simulink model "Cart_Pendulum_n9558292"  (R2018a)
settings: Solver=VariableStepAuto  StartTime=0.0  StopTime=10.0  RelTol=1e-3
model workspace (MAT data in the model file):
  F = 5
values from neighbouring files (symbols this model uses):
  g = 9.81    [MainFile_Linearised_a_n9558292.m]    (also in MainFile_Linearised_b_n9558292.m; MainFile_n9558292.m)
  l = 0.2    [MainFile_Linearised_a_n9558292.m]    (also in MainFile_Linearised_b_n9558292.m; MainFile_n9558292.m)
  m = 0.15    [MainFile_Linearised_a_n9558292.m]    (also in MainFile_Linearised_b_n9558292.m; MainFile_n9558292.m)
  Mc = 0.4    [MainFile_Linearised_a_n9558292.m]    (also in MainFile_Linearised_b_n9558292.m; MainFile_n9558292.m)
  stepf = 0.1    [MainFile_n9558292.m]
  stepi = 0    [MainFile_n9558292.m]
  stept = 1    [MainFile_n9558292.m]
  x10 = 0    [MainFile_n9558292.m]
  x20 = pi    (= 3.14159265359)    [MainFile_n9558292.m]
  x30 = 0    [MainFile_n9558292.m]
  x40 = 0    [MainFile_n9558292.m]
settings Model: Creator=haidarobeid  LastModifiedBy=haidarobeid

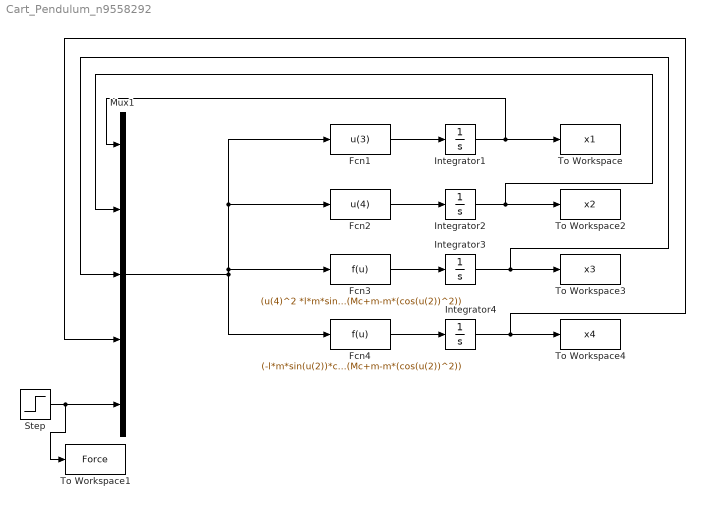
== system Cart_Pendulum_n9558292 ==
  Fcn1 : Fcn  Expr=u(3)
  Fcn2 : Fcn  Expr=u(4)
  Fcn3 : Fcn  Expr=(u(4)^2 *l*m*sin(u(2)) - g*m*sin(u(2))*cos(u(2)) +u(5))/(Mc+m-m*(cos(u(2))^2))
  Fcn4 : Fcn  Expr=(-l*m*sin(u(2))*cos(u(2))*u(4)^2 + g*(Mc+m)*sin(u(2)) - cos(u(2))*u(5) )/(Mc+m-m*(cos(u(2))^2))
  Integrator1 : Integrator  InitialCondition=x10
  Integrator2 : Integrator  InitialCondition=x20
  Integrator3 : Integrator  InitialCondition=x30
  Integrator4 : Integrator  InitialCondition=x40
  Mux1 : Mux  Inputs=5
  Step : Step  Time=stept  Before=stepi  After=stepf  SampleTime=0
  To Workspace : ToWorkspace  VariableName=x1  SampleTime=-1
  To Workspace1 : ToWorkspace  VariableName=Force  SampleTime=-1
  To Workspace2 : ToWorkspace  VariableName=x2  SampleTime=-1
  To Workspace3 : ToWorkspace  VariableName=x3  SampleTime=-1
  To Workspace4 : ToWorkspace  VariableName=x4  SampleTime=-1
  wires:
  Integrator4/1 -> Mux1/4, To Workspace4/1
  Integrator1/1 -> Mux1/1, To Workspace/1
  Integrator2/1 -> Mux1/2, To Workspace2/1
  Integrator3/1 -> Mux1/3, To Workspace3/1
  Step/1 -> To Workspace1/1, Mux1/5
  Fcn1/1 -> Integrator1/1
  Fcn2/1 -> Integrator2/1
  Fcn3/1 -> Integrator3/1
  Fcn4/1 -> Integrator4/1
  Mux1/1 -> Fcn4/1, Fcn3/1, Fcn2/1, Fcn1/1
